simulink model "exampleModel_bus_axi_w_4ptavg"  (R2017b)
settings: Solver=VariableStepAuto  StartTime=0.0  StopTime=10e-5  RelTol=1e-3
PreLoadFcn:
  | setup
values from neighbouring files (symbols this model uses):
  axiClk = 156.25e6    (= 156250000)    [setup.m]    (also in setup_exampleModel_bus_axi_simulink.m; setup_exampleModel_bus_axi_simulink_lcls2.m; setup_lcls2_pcav.m; sysgen_signal.m)
  cav1p1_addr = 204    [setup_exampleModel_bus_axi_simulink.m]    (also in setup_exampleModel_bus_axi_simulink_lcls2.m; setup_lcls2_pcav.m; sysgen_signal.m)
  cav1p2_addr = cav1p1_addr * 2    (= 408)    [setup_exampleModel_bus_axi_simulink.m]    (also in setup_exampleModel_bus_axi_simulink_lcls2.m; setup_lcls2_pcav.m; sysgen_signal.m)
  cav2p1_addr = cav1p1_addr * 3    (= 612)    [setup_exampleModel_bus_axi_simulink.m]    (also in setup_exampleModel_bus_axi_simulink_lcls2.m; setup_lcls2_pcav.m; sysgen_signal.m)
  cav2p2_addr = cav1p1_addr * 4    (= 816)    [setup_exampleModel_bus_axi_simulink.m]    (also in setup_exampleModel_bus_axi_simulink_lcls2.m; setup_lcls2_pcav.m; sysgen_signal.m)
  Fadc = Fs/interleavedChannels    (= 29750000)    [setup.m]    (also in setup_exampleModel_bus_axi_simulink.m = 357000000; setup_exampleModel_bus_axi_simulink_lcls2.m = 351000000; setup_lcls2_pcav.m = 357000000; sysgen_signal.m = 357000000)
  fir_lpf = fir1(15, w_lpf)    [setup_exampleModel_bus_axi_simulink.m]    (also in setup_exampleModel_bus_axi_simulink_lcls2.m; setup_lcls2_pcav.m)
  Fproc = 204e6    (= 204000000)    [setup_exampleModel_bus_axi_simulink.m]    (also in setup_exampleModel_bus_axi_simulink_lcls2.m = 200571400; setup_lcls2_pcav.m; sysgen_signal.m)
  Fsig = Fproc/12    (= 17000000)    [setup_exampleModel_bus_axi_simulink.m]    (also in setup_exampleModel_bus_axi_simulink_lcls2.m = 16714283.3333; setup_lcls2_pcav.m)
  Tadc = 1/fadc    (= 2.80112044818e-09)    [cavity_signal.m]    (also in setup_exampleModel_bus_axi_simulink.m; setup_exampleModel_bus_axi_simulink_lcls2.m = 2.849002849e-09; setup_lcls2_pcav.m; setup_pcav_simulink.m)
undefined symbols (not defined in the file or in its folder): AXI4, Lite
libraries: xbsIndex_r4 x2870, llrf_lib x10, simulink x3
(part 3 of 15)

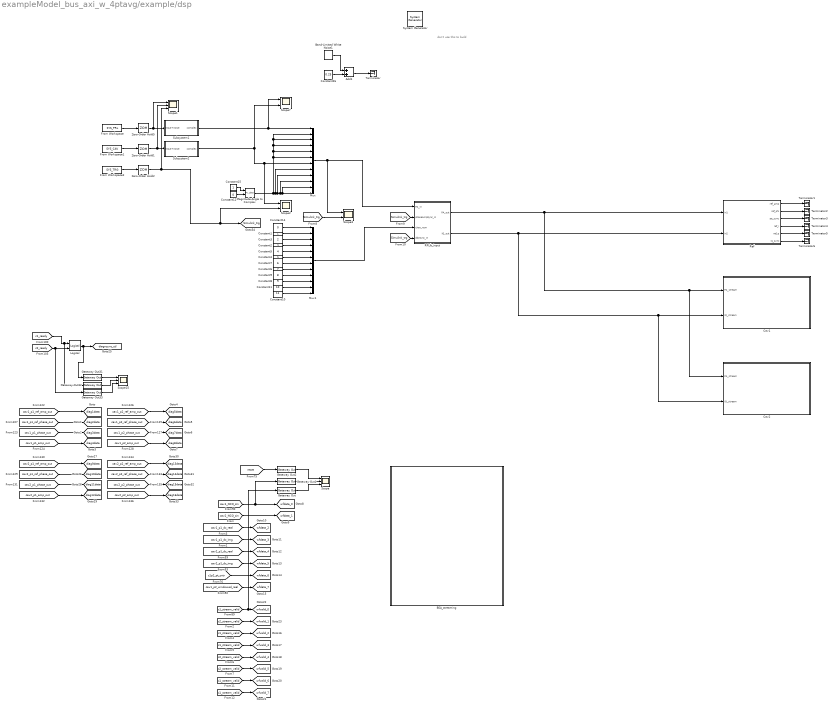
== system exampleModel_bus_axi_w_4ptavg/example/dsp ==
  note: don't use this to build
  " System Generator" : xbsIndex_r4/ System Generator  Tag=genX  xilinxfamily=kintexu  part=xcku040  speed=-2-e  package=ffva1156  synthesis_tool=Vivado  clock_wrapper=Clock Enables  directory=./netlist  proj_type=Vivado  Synth_file=Vivado Synthesis Defaults  Impl_file=Vivado Implementation Defaults  testbench=off  simulink_period=1/Fproc  sysclk_period=1e9/Fproc  dcm_input_clock_period=10  incr_netlist=off  trim_vbits=Everywhere in SubSystem  dbl_ovrd=According to Block Masks  core_generation=According to Block Masks  run_coregen=off  deprecated_control=off  eval_field=0  block_type=sysgen
  Add1 : Sum
  BSA_streaming : Subsystem
  Band-Limited White Noise1 : simulink/Sources/Band-Limited White Noise  Cov=1e-12  Ts=12/Fadc  seed=[23341]
  Cav1 : Subsystem
  Cav2 : Subsystem
  Constant1 : Constant  SampleTime=21/Fadc
  Constant10 : Constant  Value=11  SampleTime=21/Fadc
  Constant11 : Constant  Value=10  SampleTime=21/Fadc
  Constant12 : Constant  Value=0  SampleTime=21/Fadc
  Constant14 : Constant  Value=0  SampleTime=21/Fadc
  Constant15 : Constant  SampleTime=21/Fadc
  Constant2 : Constant  Value=3  SampleTime=21/Fadc
  Constant26 : Constant  Value=0.25  SampleTime=12/Fadc
  Constant3 : Constant  Value=2  SampleTime=21/Fadc
  Constant4 : Constant  Value=5  SampleTime=21/Fadc
  Constant5 : Constant  Value=4  SampleTime=21/Fadc
  Constant6 : Constant  Value=7  SampleTime=21/Fadc
  Constant7 : Constant  Value=6  SampleTime=21/Fadc
  Constant8 : Constant  Value=9  SampleTime=21/Fadc
  Constant9 : Constant  Value=8  SampleTime=21/Fadc
  From Workspace : FromWorkspace  VariableName=SYS_PRL  SampleTime=1/Fadc  OutputAfterFinalValue=Setting to zero
  From Workspace1 : FromWorkspace  VariableName=SYS_CAV  SampleTime=1/Fsig  OutputAfterFinalValue=Setting to zero
  From Workspace2 : FromWorkspace  VariableName=SYS_TRG  SampleTime=1/Fsig  OutputAfterFinalValue=Setting to zero
  Gateway Out : xbsIndex_r4/Gateway Out  inherit_from_input=off  hdl_port=on  rows=1  columns=1  UseAsDAC=off  DACChannel='1'  interface=None  automatic_assignment=on  address_offset=hex2dec('00')  intf_name=''  intf_description=''  timing_constraint=None  locs_specified=off  LOCs={}  io_standard={}  block_type=gatewayout
  Gateway Out1 : xbsIndex_r4/Gateway Out  inherit_from_input=off  hdl_port=on  rows=1  columns=1  UseAsDAC=off  DACChannel='1'  interface=None  automatic_assignment=on  address_offset=hex2dec('00')  intf_name=''  intf_description=''  timing_constraint=None  locs_specified=off  LOCs={}  io_standard={}  block_type=gatewayout
  Gateway Out2 : xbsIndex_r4/Gateway Out  inherit_from_input=off  hdl_port=on  rows=1  columns=1  UseAsDAC=off  DACChannel='1'  interface=None  automatic_assignment=on  address_offset=hex2dec('00')  intf_name=''  intf_description=''  timing_constraint=None  locs_specified=off  LOCs={}  io_standard={}  block_type=gatewayout
  Gateway Out31 : xbsIndex_r4/Gateway Out  inherit_from_input=off  hdl_port=off  rows=1  columns=1  UseAsDAC=off  DACChannel='1'  interface=None  automatic_assignment=on  address_offset=hex2dec('00')  intf_name=''  intf_description=''  timing_constraint=None  locs_specified=off  LOCs={}  io_standard={}  block_type=gatewayout
  Gateway Out32 : xbsIndex_r4/Gateway Out  inherit_from_input=off  hdl_port=off  rows=1  columns=1  UseAsDAC=off  DACChannel='1'  interface=None  automatic_assignment=on  address_offset=hex2dec('00')  intf_name=''  intf_description=''  timing_constraint=None  locs_specified=off  LOCs={}  io_standard={}  block_type=gatewayout
  Gateway Out33 : xbsIndex_r4/Gateway Out  inherit_from_input=off  hdl_port=off  rows=1  columns=1  UseAsDAC=off  DACChannel='1'  interface=None  automatic_assignment=on  address_offset=hex2dec('00')  intf_name=''  intf_description=''  timing_constraint=None  locs_specified=off  LOCs={}  io_standard={}  block_type=gatewayout
  Logical : xbsIndex_r4/Logical  logical_function=AND  inputs=2  en=off  latency=1  precision=Full  arith_type=Unsigned  n_bits=16  bin_pt=0  align_bp=on  dbl_ovrd=off  block_type=logical
  Magnitude-Angle to Complex : MagnitudeAngleToComplex
  Mux : Mux  Inputs=12
  Mux1 : Mux  Inputs=12
  RFLib_input : Subsystem
  Ref : Subsystem
  Scope : Scope  NumInputPorts=3
  Scope1 : Scope  NumInputPorts=3
  Scope15 : Scope  NumInputPorts=3
  Scope2 : Scope  NumInputPorts=2
  Scope3 : Scope  NumInputPorts=2
  Scope7 : Scope  NumInputPorts=2
  Subsystem1 : Subsystem
  Subsystem2 : Subsystem
  Terminator{,1..6} (7 alike) : Terminator
  Zero-Order Hold1 : ZeroOrderHold  SampleTime=1/Fadc
  Zero-Order Hold2 : ZeroOrderHold  SampleTime=1/Fadc
  Zero-Order Hold5 : ZeroOrderHold  SampleTime=1/Fadc
  tag scope: Simulink_trg=global, diag10data=global, diag11data=global, diag12data=global, diag13data=global, diag14data=global, diag15data=global, diag16data=global, diag1data=global, diag2data=global, diag3data=global, diag4data=global, diag5data=global, diag6data=global, diag7data=global, diag8data=global, diag9data=global, diagnsync_ctl=global, wfdata_0=global, wfdata_1=global, wfdata_2=global, wfdata_3=global, wfdata_4=global, wfdata_5=global, wfdata_6=global, wfdata_7=global, wfvalid_0=global, wfvalid_1=global, wfvalid_2=global, wfvalid_3=global, wfvalid_4=global, wfvalid_5=global, wfvalid_6=global, wfvalid_7=global
  wires:
  Constant14/1 -> Mux1/1
  From Workspace1/1 -> Zero-Order Hold1/1
  Band-Limited White Noise1/1 -> Add1/1
  Constant26/1 -> Add1/2
  From Workspace/1 -> Zero-Order Hold5/1
  Add1/1 -> Terminator/1
  Constant1/1 -> Mux1/2
  Constant2/1 -> Mux1/4
  Constant3/1 -> Mux1/3
  Constant7/1 -> Mux1/7
  Constant6/1 -> Mux1/8
  Constant4/1 -> Mux1/6
  Constant5/1 -> Mux1/5
  Constant9/1 -> Mux1/9
  Constant8/1 -> Mux1/10
  Constant10/1 -> Mux1/12
  Constant11/1 -> Mux1/11
  Zero-Order Hold1/1 -> Scope1/2, Subsystem2/1(input+noise)
  Subsystem1/1(complex) -> Scope7/1, Mux/1
  Subsystem2/1(complex) -> Scope2/1, Mux/7, Scope7/2
  RFLib_input/2(IQ_out) -> Cav2/2(IQ_stream), Cav1/2(IQ_stream), Ref/2(In2)
  RFLib_input/1(PA_out) -> Ref/1(In1), Cav2/1(PA_stream), Cav1/1(PA_stream)
  Mux/1 -> Scope3/1, RFLib_input/1(PA_in)
  Mux1/1 -> RFLib_input/3(chan_num)
  Magnitude-Angle to Complex/1 -> Mux/2, Mux/3, Mux/4, Mux/5, Mux/6, Mux/8, Mux/9, Mux/10, Mux/11, Mux/12
  Constant12/1 -> Magnitude-Angle to Complex/2
  Constant15/1 -> Magnitude-Angle to Complex/1
  [c1_stream_valid] -> [wfvalid_7]
  [cav1_NCO_sin] -> Gateway Out1/1, [wfdata_0]
  [cav2_p1_dc_img] -> [wfdata_5]
  [c1p2_pt_cntr] -> [wfdata_6]
  [c2_stream_valid] -> [wfvalid_1]
  [cav2_p1_dc_real] -> [wfdata_4]
  [c1_stream_valid] -> [wfvalid_6]
  [c1_stream_valid] -> Gateway Out/1, [wfvalid_0]
  [c1_stream_valid] -> [wfvalid_3]
  [cav1_p2_windowed_real] -> [wfdata_7]
  [cav1_p1_dc_img] -> [wfdata_3]
  [cav1_p1_dc_real] -> [wfdata_2]
  [cav2_NCO_sin] -> [wfdata_1]
  [c2_stream_valid] -> [wfvalid_4]
  [c2_stream_valid] -> [wfvalid_5]
  [c1_stream_valid] -> [wfvalid_2]
  Ref/1(ref_amp) -> Terminator1/1
  Ref/2(ref_phi) -> Terminator2/1
  Ref/3(pa_sync) -> Terminator3/1
  Ref/4(ref_i) -> Terminator4/1
  Ref/5(ref_q) -> Terminator5/1
  Ref/6(iq_sync) -> Terminator6/1
  Zero-Order Hold5/1 -> Scope1/1, Subsystem1/1(input+noise)
  [c1_ready] -> Gateway Out32/1, Logical/1
  Gateway Out32/1 -> Scope15/2
  Gateway Out31/1 -> Scope15/1
  Logical/1 -> Gateway Out31/1, [diagnsync_ctl]
  Gateway Out33/1 -> Scope15/3
  [c2_ready] -> Gateway Out33/1, Logical/2
  [cav1_p1_ref_amp_out] -> [diag1data]
  [cav1_p1_ref_phase_out] -> [diag2data]
  [cav1_p1_phase_out] -> [diag3data]
  [cav1_p1_amp_out] -> [diag4data]
  [cav1_p2_ref_amp_out] -> [diag5data]
  [cav1_p2_ref_phase_out] -> [diag6data]
  [cav1_p2_phase_out] -> [diag7data]
  [cav1_p2_amp_out] -> [diag8data]
  [cav2_p1_ref_amp_out] -> [diag9data]
  [cav2_p1_ref_phase_out] -> [diag10data]
  [cav2_p1_phase_out] -> [diag11data]
  [cav2_p1_amp_out] -> [diag12data]
  [cav2_p2_ref_amp_out] -> [diag13data]
  [cav2_p2_ref_phase_out] -> [diag14data]
  [cav2_p2_phase_out] -> [diag15data]
  [cav2_p2_amp_out] -> [diag16data]
  From Workspace2/1 -> Zero-Order Hold2/1
  Zero-Order Hold2/1 -> [Simulink_trg], Scope2/2, Scope1/3
  [Simulink_trg] -> Scope3/2
  [Simulink_trg] -> RFLib_input/4(ddcSync_in)
  [Simulink_trg] -> RFLib_input/2(phaseAmpSync_in)
  Gateway Out1/1 -> Scope/2
  Gateway Out/1 -> Scope/3
  Gateway Out2/1 -> Scope/1
  [reset] -> Gateway Out2/1
